simulink model "scattering_based_force_vel"  (R2020b)
settings: Solver=ode45  StartTime=0.0  StopTime=10  RelTol=1e-3
values from neighbouring files (symbols this model uses):
  A = [1 Ts ... (first row only)    [hw6_main_force_vel.m]    (also in hw6_main_fv_kalman.m; hw6_new.m)
  Amp = 1    [hw6_main_force_vel.m]    (also in hw6_main_fv.m = 0.8; hw6_main_fv_kalman.m = 0.8; hw6_new.m)
  b = 1    [hw6_main_force_vel.m]    (also in hw6_main_fv.m; hw6_main_fv_kalman.m; hw6_new.m)
  Be = 10    [hw6_main_force_vel.m]    (also in hw6_main_fv.m = 20; hw6_main_fv_kalman.m = 20; hw6_new.m)
  Bh = 70    [hw6_main_force_vel.m]    (also in hw6_main_fv.m = 1.5; hw6_main_fv_kalman.m = 1.5; hw6_new.m = 0)
  Bs = 100    [hw6_main_force_vel.m]    (also in hw6_main_fv.m; hw6_main_fv_kalman.m = 50; hw6_new.m = 600)
  C = [1 0]    [hw6_main_force_vel.m]    (also in hw6_main_fv_kalman.m; hw6_new.m)
  delay = 1    [hw6_main_force_vel.m]    (also in hw6_main_fv.m = 10; hw6_main_fv_kalman.m = 10; hw6_new.m)
  Dh = 700    [hw6_main_force_vel.m]    (also in hw6_main_fv.m = 8; hw6_main_fv_kalman.m = 8; hw6_new.m = 10)
  Dm = 5    [hw6_main_force_vel.m]    (also in hw6_main_fv.m = 0; hw6_main_fv_kalman.m = 0; hw6_new.m = 4)
  Ds = 0    [hw6_main_force_vel.m]    (also in hw6_main_fv.m; hw6_main_fv_kalman.m; hw6_new.m = 50)
  Fc = 1    [hw6_main_force_vel.m]    (also in hw6_main_fv.m = 0.1; hw6_new.m = 0.5)
  Fip = 10    [hw6_main_force_vel.m]    (also in hw6_main_fv.m = 5; hw6_new.m = 100)
  Je = 0    [hw6_main_force_vel.m]    (also in hw6_main_fv.m; hw6_main_fv_kalman.m; hw6_new.m)
  Jh = 1    [hw6_main_force_vel.m]    (also in hw6_main_fv.m = 0; hw6_main_fv_kalman.m = 0; hw6_new.m = 0)
  Ke = 200    [hw6_main_force_vel.m]    (also in hw6_main_fv.m = 210; hw6_main_fv_kalman.m = 210; hw6_new.m = 10)
  Kh = 2000    [hw6_main_force_vel.m]    (also in hw6_main_fv.m = 1; hw6_main_fv_kalman.m = 0.1; hw6_new.m = 1)
  Ks = 0    [hw6_main_force_vel.m]    (also in hw6_main_fv.m = 80; hw6_main_fv_kalman.m = 60; hw6_new.m = 800)
  Mm = 0.5    [hw6_main_force_vel.m]    (also in hw6_main_fv.m; hw6_main_fv_kalman.m; hw6_new.m = 2)
  Ms = 2    [hw6_main_force_vel.m]    (also in hw6_main_fv.m; hw6_main_fv_kalman.m; hw6_new.m = 40)
  Ph = 13000    [hw6_main_force_vel.m]    (also in hw6_main_fv.m = 1; hw6_main_fv_kalman.m = 1; hw6_new.m = 1)
  posNoiseVar = 0.0001    [hw6_main_force_vel.m]    (also in hw6_main_fv_kalman.m; hw6_new.m = 1e-05)
  R_m = 1    [hw6_main_force_vel.m]    (also in hw6_main_fv_kalman.m; hw6_new.m)
  R_s = 1    [hw6_main_force_vel.m]    (also in hw6_main_fv_kalman.m; hw6_new.m)
  torqueNoiseVar = 0.000    (= 0)    [hw6_main_force_vel.m]    (also in hw6_main_fv_kalman.m = 0.01; hw6_new.m = 0.01)
  Ts = 0.001    [hw6_main_force_vel.m]    (also in hw6_main_fv.m; hw6_main_fv_kalman.m; hw6_new.m)
  xe = 4    [hw6_main_force_vel.m]    (also in hw6_main_fv.m = 0.5; hw6_main_fv_kalman.m = 0.5; hw6_new.m = 1.5)
undefined symbols (not defined in the file or in its folder): DiscIntNeverNeededParam, Discrete, Time
libraries: simulink x4, ctrlSharedLib x2
settings Model: Creator=nicol  LastModifiedBy=nicol

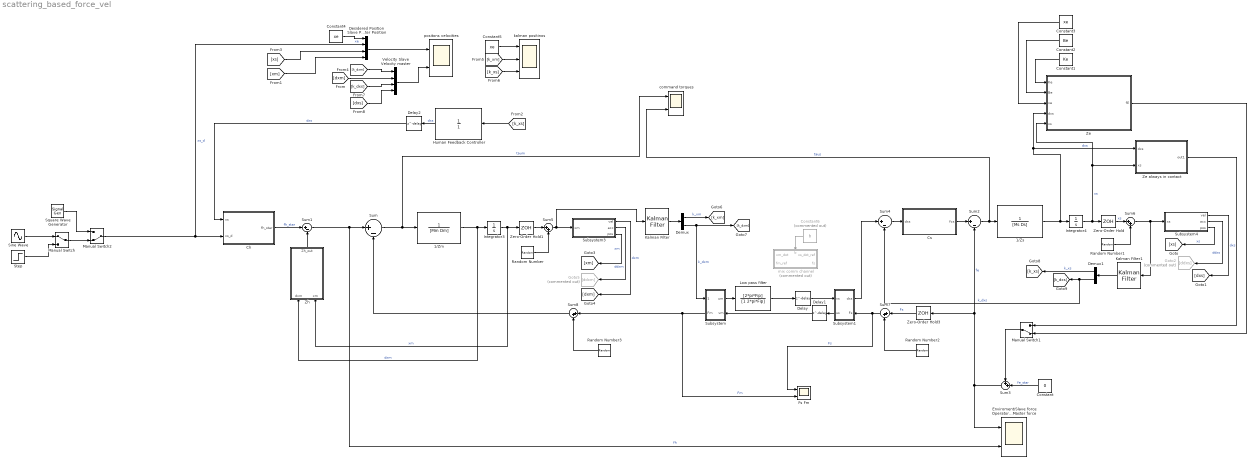
== system scattering_based_force_vel ==
  1/Zm : TransferFcn  Denominator=[Mm Dm]
  1/Zs : TransferFcn  Denominator=[Ms Ds]
  Ch : Subsystem
  Constant : Constant  Value=0
  Constant1 : Constant  Value=Ke
  Constant2 : Constant  Value=Be
  Constant3 : Constant  Value=xe
  Constant4 : Constant  Value=xe
  Constant5 : Constant  Value=xe
  Constant6 : Constant  Commented=on  Value=b
  Cs : Subsystem
  Delay : Delay  DelayLength=delay  SampleTime=Ts
  Delay1 : Delay  DelayLength=delay  SampleTime=Ts
  Delay2 : Delay  DelayLength=delay  SampleTime=Ts
  Demux : Demux  Outputs=2
  Demux1 : Demux  Outputs=2
  Desidered Position Slave Position Master Position : Mux
  Enviroment/Slave force Operator/Master force : Scope  NumInputPorts=2
  Fs Fm : Scope  NumInputPorts=2
  Goto2 : Goto  Commented=on  GotoTag=ddxs
  Goto5 : Goto  Commented=on  GotoTag=ddxm
  Human Feedback Controller : TransferFcn  Denominator=[1]
  Integrator3 : Integrator
  Integrator4 : Integrator
  Kalman Filter : ctrlSharedLib/Kalman Filter  TimeDomain=Discrete-Time  UseCurrentEstimator=on  ModelSource=Individual A, B, C, D matrices  ModelSourceVariable=ss(0.95,1,0,0,Ts)  A=A  B=1  C=C  D=0  NumberOfStates=1  NumberOfInputs=1  NumberOfOutputs=1  InitialEstimateSource=Dialog  X0=0  P0=10  UseK=off  UseGH=off  NumberOfProcessNoiseInputs=1  G=1  TimeInvariantG=on  H=0  TimeInvariantH=on  Q=Q_m  TimeInvariantQ=on  R=R_m  TimeInvariantR=on  N=0  TimeInvariantN=on  AddInputPort=off  AddEnablePort=off  OutputEstimatedY=off  OutputP=off  Ts=Ts
  Kalman Filter1 : ctrlSharedLib/Kalman Filter  TimeDomain=Discrete-Time  UseCurrentEstimator=on  ModelSource=Individual A, B, C, D matrices  ModelSourceVariable=ss(0.95,1,0,0,Ts)  A=A  B=1  C=C  D=0  NumberOfStates=1  NumberOfInputs=1  NumberOfOutputs=1  InitialEstimateSource=Dialog  X0=0  P0=10  UseK=off  UseGH=off  NumberOfProcessNoiseInputs=1  G=1  TimeInvariantG=on  H=0  TimeInvariantH=on  Q=Q_s  TimeInvariantQ=on  R=R_s  TimeInvariantR=on  N=0  TimeInvariantN=on  AddInputPort=off  AddEnablePort=off  OutputEstimatedY=off  OutputP=off  Ts=Ts
  Low pass filter : TransferFcn  Numerator=[2*pi*Fip]  Denominator=[1 2*pi*Fip]
  Manual Switch : ManualSwitch
  Manual Switch1 : ManualSwitch  CurrentSetting=0
  Manual Switch2 : ManualSwitch  CurrentSetting=0
  Random Number : RandomNumber  Variance=posNoiseVar  SampleTime=Ts
  Random Number1 : RandomNumber  Variance=posNoiseVar  SampleTime=Ts
  Random Number2 : RandomNumber  Variance=torqueNoiseVar  SampleTime=Ts
  Random Number3 : RandomNumber  Variance=torqueNoiseVar  SampleTime=Ts
  Sine Wave : Sin  Amplitude=Amp  Frequency=2*pi*Fc  SampleTime=0
  Square Wave Generator : SignalGenerator  WaveForm=square  Amplitude=Amp  Frequency=Fc  Units=rad/sec
  Step : Step  Time=Amp  SampleTime=0
  Subsystem : Subsystem
      settings: PortSchema="{\"entries\":[{\"content\":{\"sides\":[{\"content\":{\"connectorIds\":[\"In1\",\"Out2\"]},\"type\":\"ConnectorPlacement.EquallySpacedRectSide\",\"uuid\":\"82be490b-f4e1-4469-8bd6-488a0e070f91\"},{\"content\":{\"connectorIds\":[\"Out1\",\"In2\"],\"side\":\"RIGHT\"},\"type\":\"ConnectorPlacement.EquallySpacedRectSide\",\"uuid\":\"c4a13bf6-21c5-475e-be70-cb3636e820b8\"},{\"content\":{\"connectorIds\":[],\"side\":\"TOP\"},\"type\":\"ConnectorPlacement.EquallySpacedRectSide\",\"uuid\":\"239945ea-98d9-43ca-9337-d0acd489fa2c\"},{\"content\":{\"connectorIds\":[],\"side\":\"HIDDEN\"},\"type\":\"ConnectorPlacement.EquallySpacedRectSide\",\"uuid\":\"ab55d6c9-2d6b-496a-b62d-f74546630c92\"}]},\"type\":\"ConnectorPlacement.EquallySpacedConnector\",\"uuid\":\"f2ee4140-76ed-4153-9f7f-3580e67d072a\"}],\"packageUris\":[\"http://schema.mathworks.com/mf0/Connector/R2020b\"],\"version\":\"1.0\"}"
  Subsystem1 : Subsystem
      settings: PortSchema="{\"entries\":[{\"content\":{\"sides\":[{\"content\":{\"connectorIds\":[\"In1\",\"Out2\"]},\"type\":\"ConnectorPlacement.EquallySpacedRectSide\",\"uuid\":\"82be490b-f4e1-4469-8bd6-488a0e070f91\"},{\"content\":{\"connectorIds\":[\"Out1\",\"In2\"],\"side\":\"RIGHT\"},\"type\":\"ConnectorPlacement.EquallySpacedRectSide\",\"uuid\":\"c4a13bf6-21c5-475e-be70-cb3636e820b8\"},{\"content\":{\"connectorIds\":[],\"side\":\"TOP\"},\"type\":\"ConnectorPlacement.EquallySpacedRectSide\",\"uuid\":\"239945ea-98d9-43ca-9337-d0acd489fa2c\"},{\"content\":{\"connectorIds\":[],\"side\":\"HIDDEN\"},\"type\":\"ConnectorPlacement.EquallySpacedRectSide\",\"uuid\":\"ab55d6c9-2d6b-496a-b62d-f74546630c92\"}]},\"type\":\"ConnectorPlacement.EquallySpacedConnector\",\"uuid\":\"f2ee4140-76ed-4153-9f7f-3580e67d072a\"}],\"packageUris\":[\"http://schema.mathworks.com/mf0/Connector/R2020b\"],\"version\":\"1.0\"}"
  Subsystem3 : Subsystem
  Subsystem4 : Subsystem
  Sum{,1..2,4} (4 alike) : Sum  Inputs=|+-
  Sum3 : Sum  Inputs=++|
  Sum{5..8} (4 alike) : Sum  Inputs=|++
  Velocity Slave Velocity master : Mux
  Ze : MATLAB Function  TreatAsAtomicUnit=on
  Ze always in contact : Subsystem
  Zero-Order Hold : ZeroOrderHold  SampleTime=Ts
  Zero-Order Hold1 : ZeroOrderHold  SampleTime=Ts
  Zero-Order Hold3 : ZeroOrderHold  SampleTime=Ts
  Zh : Subsystem
  command torques : Scope  NumInputPorts=2
  kalman positinos : Scope  NumInputPorts=3
  mix comm channel : Subsystem  Commented=on
      settings: PortSchema="{\"entries\":[{\"content\":{\"sides\":[{\"content\":{\"connectorIds\":[\"In1\",\"Out2\"]},\"type\":\"ConnectorPlacement.EquallySpacedRectSide\",\"uuid\":\"bc86f248-d301-4246-9174-3009eb7a28c8\"},{\"content\":{\"connectorIds\":[\"Out1\",\"In3\"],\"side\":\"RIGHT\"},\"type\":\"ConnectorPlacement.EquallySpacedRectSide\",\"uuid\":\"557cd81f-37dd-4057-aedb-d298233d4d9a\"},{\"content\":{\"connectorIds\":[\"In2\"],\"side\":\"TOP\"},\"type\":\"ConnectorPlacement.EquallySpacedRectSide\",\"uuid\":\"3402ae9d-bb8b-45e3-a665-d7336455e600\"},{\"content\":{\"connectorIds\":[],\"side\":\"HIDDEN\"},\"type\":\"ConnectorPlacement.EquallySpacedRectSide\",\"uuid\":\"007c7815-feca-4fba-aeae-7d69e2449b19\"}]},\"type\":\"ConnectorPlacement.EquallySpacedConnector\",\"uuid\":\"a34d2d5f-5fa4-4153-a6c8-331f90676310\"}],\"packageUris\":[\"http://schema.mathworks.com/mf0/Connector/R2020b\"],\"version\":\"1.0\"}"
  "positons velocities " : Scope  NumInputPorts=2
  wires:
  Ch/1(fh_star) -> Sum1/1  "fh_star"
  Zh/1(Zh_out) -> Sum1/2
  1/Zm/1 -> Zh/1(dxm), Integrator3/1  "dxm"
  Sum1/1 -> Enviroment/Slave force Operator/Master force/2, Sum/1  "fh"
  Cs/1(fcs) -> Sum2/1
  1/Zs/1 -> Integrator4/1, Ze always in contact/1(dxs), Ze/4(dxs)  "dxs"
  Sum2/1 -> 1/Zs/1, command torques/2  "taus"
  Ze/1(fE) -> Manual Switch1/2
  Sum3/1 -> Enviroment/Slave force Operator/Master force/1, Zero-Order Hold3/1, Sum2/2  "fe"
  Constant/1 -> Sum3/2  "fe_star"
  Constant1/1 -> Ze/1(Ke)
  Constant2/1 -> Ze/2(Be)
  Constant3/1 -> Ze/3(xe)
  Integrator4/1 -> Zero-Order Hold/1, Ze/5(xs), Ze always in contact/2(xs)  "xs"
  Manual Switch1/1 -> Sum3/1
  Ze always in contact/1(out1) -> Manual Switch1/1
  Sum/1 -> command torques/1, 1/Zm/1  "taum"
  Velocity Slave Velocity master/1 -> "positons velocities "/2
  Desidered Position Slave Position Master Position/1 -> "positons velocities "/1
  Sum4/1 -> Cs/1(dxs)
  Manual Switch2/1 -> Desidered Position Slave Position Master Position/2, Ch/2(xs_d)  "xs_d"
  Subsystem3/1(vel) -> [dxm]  "dxm"
  Subsystem3/3(pos) -> [xm]  "xm"
  Integrator3/1 -> Zero-Order Hold1/1, Zh/2(xm)  "xm"
  Subsystem3/2(acc) -> Goto5/1  "ddxm"
  Zero-Order Hold1/1 -> Sum5/1
  Subsystem4/2(acc) -> Goto2/1  "ddxs"
  Subsystem4/1(vel) -> [dxs]  "dxs"
  Subsystem4/3(pos) -> [xs]  "xs"
  Zero-Order Hold/1 -> Sum6/1  "xs"
  [k_xs] -> Human Feedback Controller/1
  Delay2/1 -> Ch/1(xs)  "dxs"
  Square Wave Generator/1 -> Manual Switch2/1
  Delay1/1 -> Subsystem/2(vm)
  Delay/1 -> Subsystem1/1(vs)
  Subsystem/1(um) -> Low pass filter/1
  Subsystem1/2(us) -> Delay1/1
  Zero-Order Hold3/1 -> Sum7/1  "Fs"
  Human Feedback Controller/1 -> Delay2/1  "dxs"
  Sum5/1 -> Kalman Filter/1, Subsystem3/1(xm)
  Random Number/1 -> Sum5/2
  Random Number1/1 -> Sum6/2
  Sum6/1 -> Kalman Filter1/1, Subsystem4/1(xs)
  Sum7/1 -> Subsystem1/2(Fs), Fs Fm/1  "Fs"
  Random Number2/1 -> Sum7/2
  Sum8/1 -> Sum/2
  Random Number3/1 -> Sum8/2
  Sine Wave/1 -> Manual Switch/1
  Kalman Filter/1 -> Demux/1
  Demux/1 -> [k_xm]  "k_xm"
  [dxm] -> Velocity Slave Velocity master/2
  [xm] -> Desidered Position Slave Position Master Position/4
  [xs] -> Desidered Position Slave Position Master Position/3
  Demux/2 -> [k_dxm], Subsystem/1(dxm)  "k_dxm"
  [k_dxm] -> Velocity Slave Velocity master/1
  Kalman Filter1/1 -> Demux1/1
  Demux1/2 -> Sum4/2, [k_dxs]  "k_dxs"
  Demux1/1 -> [k_xs]  "k_xs"
  [k_dxs] -> Velocity Slave Velocity master/3
  [k_xm] -> kalman positinos/2
  [k_xs] -> kalman positinos/3
  Constant4/1 -> Desidered Position Slave Position Master Position/1  "xe"
  Constant5/1 -> kalman positinos/1
  Constant6/1 -> mix comm channel/2(b)
  Subsystem/2(Fm) -> Fs Fm/2, Sum8/1  "Fm"
  Subsystem1/1(dxs) -> Sum4/1
  Low pass filter/1 -> Delay/1
  [dxs] -> Velocity Slave Velocity master/4
  Manual Switch/1 -> Manual Switch2/2
  Step/1 -> Manual Switch/2

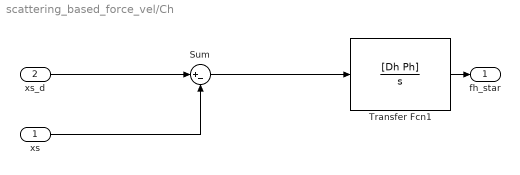
== system scattering_based_force_vel/Ch ==
  xs : Inport
  xs_d : Inport  Port=2
  Sum : Sum  Inputs=|+-
  Transfer Fcn1 : TransferFcn  Numerator=[Dh Ph]  Denominator=[1 0]
  fh_star : Outport
  wires:
  xs/1 -> Sum/2
  Sum/1 -> Transfer Fcn1/1
  Transfer Fcn1/1 -> fh_star/1
  xs_d/1 -> Sum/1

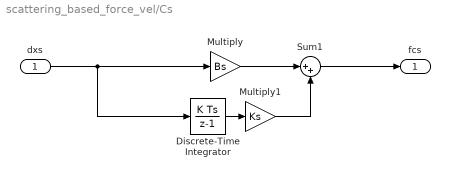
== system scattering_based_force_vel/Cs ==
  dxs : Inport
  Discrete-Time Integrator : DiscreteIntegrator  SampleTime=-1  ICPrevOutput=DiscIntNeverNeededParam  ICPrevScaledInput=DiscIntNeverNeededParam
  Multiply : Gain  Gain=Bs
  Multiply1 : Gain  Gain=Ks
  Sum1 : Sum  Inputs=|++
  fcs : Outport
  wires:
  dxs/1 -> Discrete-Time Integrator/1, Multiply/1
  Multiply1/1 -> Sum1/2
  Multiply/1 -> Sum1/1
  Sum1/1 -> fcs/1
  Discrete-Time Integrator/1 -> Multiply1/1

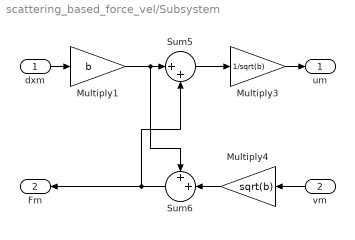
== system scattering_based_force_vel/Subsystem ==
  dxm : Inport
  vm : Inport  Port=2
  Multiply1 : Gain  Gain=b
  Multiply3 : Gain  Gain=1/sqrt(b)
  Multiply4 : Gain  Gain=sqrt(b)
  Sum5 : Sum  Inputs=|++
  Sum6 : Sum  Inputs=++|
  um : Outport
  Fm : Outport  Port=2
  wires:
  Sum6/1 -> Fm/1, Sum5/2
  Multiply1/1 -> Sum6/1, Sum5/1
  Sum5/1 -> Multiply3/1
  Multiply4/1 -> Sum6/2
  vm/1 -> Multiply4/1
  Multiply3/1 -> um/1
  dxm/1 -> Multiply1/1

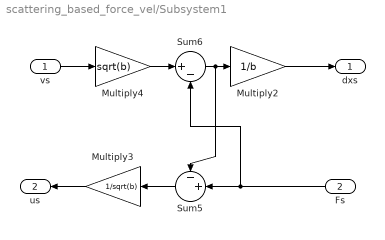
== system scattering_based_force_vel/Subsystem1 ==
  vs : Inport
  Fs : Inport  Port=2
  Multiply2 : Gain  Gain=1/b
  Multiply3 : Gain  Gain=1/sqrt(b)
  Multiply4 : Gain  Gain=sqrt(b)
  Sum5 : Sum  Inputs=-+|
  Sum6 : Sum  Inputs=|+-
  dxs : Outport
  us : Outport  Port=2
  wires:
  Sum6/1 -> Sum5/1, Multiply2/1
  Sum5/1 -> Multiply3/1
  Fs/1 -> Sum5/2, Sum6/2
  vs/1 -> Multiply4/1
  Multiply2/1 -> dxs/1
  Multiply3/1 -> us/1
  Multiply4/1 -> Sum6/1

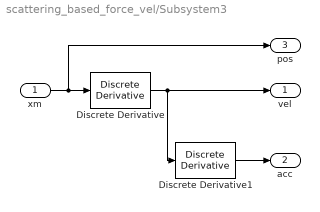
== system scattering_based_force_vel/Subsystem3 ==
  xm : Inport
  Discrete Derivative : simulink/Discrete/Discrete Derivative  gainval=1.0  ICPrevScaledInput=0.0  OutMin=[]  OutMax=[]  OutDataType=fixdt(1, 16)  OutScaling=2^-10  DoSatur=off
  Discrete Derivative1 : simulink/Discrete/Discrete Derivative  gainval=1.0  ICPrevScaledInput=0.0  OutMin=[]  OutMax=[]  OutDataType=fixdt(1, 16)  OutScaling=2^-10  DoSatur=off
  vel : Outport
  acc : Outport  Port=2
  pos : Outport  Port=3
  wires:
  xm/1 -> pos/1, Discrete Derivative/1
  Discrete Derivative/1 -> Discrete Derivative1/1, vel/1
  Discrete Derivative1/1 -> acc/1

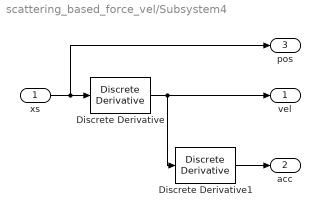
== system scattering_based_force_vel/Subsystem4 ==
  xs : Inport
  Discrete Derivative : simulink/Discrete/Discrete Derivative  gainval=1.0  ICPrevScaledInput=0.0  OutMin=[]  OutMax=[]  OutDataType=fixdt(1, 16)  OutScaling=2^-10  DoSatur=off
  Discrete Derivative1 : simulink/Discrete/Discrete Derivative  gainval=1.0  ICPrevScaledInput=0.0  OutMin=[]  OutMax=[]  OutDataType=fixdt(1, 16)  OutScaling=2^-10  DoSatur=off
  vel : Outport
  acc : Outport  Port=2
  pos : Outport  Port=3
  wires:
  xs/1 -> pos/1, Discrete Derivative/1
  Discrete Derivative/1 -> Discrete Derivative1/1, vel/1
  Discrete Derivative1/1 -> acc/1

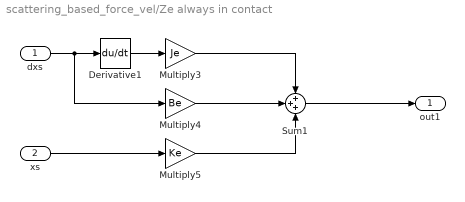
== system scattering_based_force_vel/Ze always in contact ==
  dxs : Inport
  xs : Inport  Port=2
  Derivative1 : Derivative
  Multiply3 : Gain  Gain=Je
  Multiply4 : Gain  Gain=Be
  Multiply5 : Gain  Gain=Ke
  Sum1 : Sum  Inputs=+++
  out1 : Outport
  wires:
  Sum1/1 -> out1/1
  Multiply4/1 -> Sum1/2
  Multiply5/1 -> Sum1/3
  dxs/1 -> Multiply4/1, Derivative1/1
  Derivative1/1 -> Multiply3/1
  xs/1 -> Multiply5/1
  Multiply3/1 -> Sum1/1

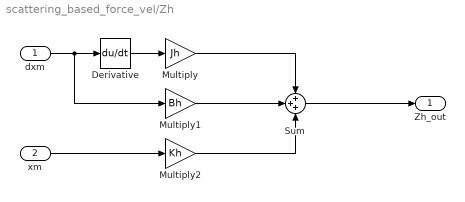
== system scattering_based_force_vel/Zh ==
  dxm : Inport
  xm : Inport  Port=2
  Derivative : Derivative
  Multiply : Gain  Gain=Jh
  Multiply1 : Gain  Gain=Bh
  Multiply2 : Gain  Gain=Kh
  Sum : Sum  Inputs=+++
  Zh_out : Outport
  wires:
  dxm/1 -> Multiply1/1, Derivative/1
  Derivative/1 -> Multiply/1
  Sum/1 -> Zh_out/1
  xm/1 -> Multiply2/1
  Multiply1/1 -> Sum/2
  Multiply/1 -> Sum/1
  Multiply2/1 -> Sum/3

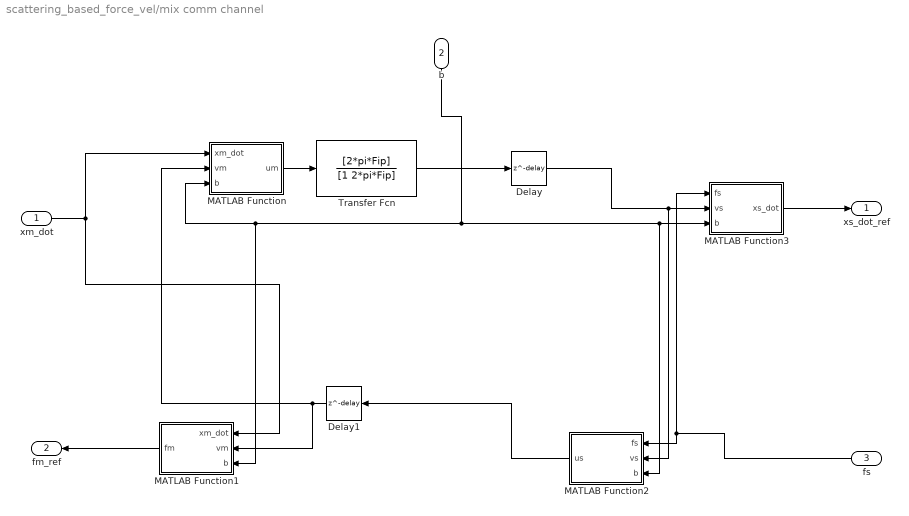
== system scattering_based_force_vel/mix comm channel ==
  xm_dot : Inport
  b : Inport  Port=2
  fs : Inport  Port=3
  Delay : Delay  DelayLength=delay  SampleTime=Ts
  Delay1 : Delay  DelayLength=delay  SampleTime=Ts
  MATLAB Function : MATLAB Function  TreatAsAtomicUnit=on
  MATLAB Function1 : MATLAB Function  TreatAsAtomicUnit=on
  MATLAB Function2 : MATLAB Function  TreatAsAtomicUnit=on
  MATLAB Function3 : MATLAB Function  TreatAsAtomicUnit=on
  Transfer Fcn : TransferFcn  Numerator=[2*pi*Fip]  Denominator=[1 2*pi*Fip]
  xs_dot_ref : Outport
  fm_ref : Outport  Port=2
  wires:
  b/1 -> MATLAB Function1/3(b), MATLAB Function/3(b), MATLAB Function2/3(b), MATLAB Function3/3(b)
  xm_dot/1 -> MATLAB Function1/1(xm_dot), MATLAB Function/1(xm_dot)
  MATLAB Function1/1(fm) -> fm_ref/1
  fs/1 -> MATLAB Function3/1(fs), MATLAB Function2/1(fs)
  MATLAB Function3/1(xs_dot) -> xs_dot_ref/1
  MATLAB Function/1(um) -> Transfer Fcn/1
  Delay/1 -> MATLAB Function2/2(vs), MATLAB Function3/2(vs)
  Delay1/1 -> MATLAB Function/2(vm), MATLAB Function1/2(vm)
  Transfer Fcn/1 -> Delay/1
  MATLAB Function2/1(us) -> Delay1/1

== matlab function scattering_based_force_vel/Ze ==
  data: Ke input; fE output; Be input; xe input; dxs input; xs input
function fE = environment(Ke,Be,xe,dxs,xs)
if(xs>xe)
    fE=Ke*(xs-xe)+Be*dxs;
else
    fE=0;
end

== matlab function scattering_based_force_vel/mix comm channel/MATLAB Function ==
  data: xm_dot input; um output; vm input; b input
function um = fcn(xm_dot, vm, b)

um = sqrt(2*b)*xm_dot+vm;

== matlab function scattering_based_force_vel/mix comm channel/MATLAB Function1 ==
  data: xm_dot input; fm output; vm input; b input
function fm = fcn(xm_dot, vm, b)

fm = b*xm_dot+sqrt(2*b)*vm;

== matlab function scattering_based_force_vel/mix comm channel/MATLAB Function2 ==
  data: fs input; us output; vs input; b input
function us = fcn(fs, vs, b)

us = sqrt(2/b)*fs-vs;

== matlab function scattering_based_force_vel/mix comm channel/MATLAB Function3 ==
  data: fs input; xs_dot output; vs input; b input
function xs_dot = fcn(fs, vs, b)

xs_dot = -1/b*(fs-sqrt(2*b)*vs);
